simulink model "vector_vehicle_canoe"  (Simulink 7.7)
settings: Solver=ode3  StartTime=0.0  StopTime=10.0  FixedStep=T  RelTol=1e-3
libraries: canoelib x70, simulink x3
settings Model: Creator=vismso  LastModifiedBy=visjf
settings DataIOCC: SaveOutput=off  SignalLogging=off  SaveTime=off
settings OptimizationCC: InlineParams=on  UseIntDivNetSlope=on  SimCompilerOptimization=On
settings DebuggingCC: ArtificialAlgebraicLoopMsg=none  StrictBusMsg=Warning
settings RTWCC: SystemTargetFile=cn.tlc  TemplateMakefile=cn_msdll.tmf  Description=Vector CANoe Real-Time Target DLL (Visual C/C++ Project Makefile)  ProcessScript=cn_make_rtw_hook
settings CodeAppCC: MaxIdLength=128
settings STFCustomTargetCC: FunctionExecutionProfile=off  GeneratePreprocessorConditionals=Disable all  MatFileLogging=on  SystemTargetFile=cn.tlc
settings GRTTargetCC: ParMdlRefBuildCompliant=off  CompOptLevelCompliant=off  ExtModeMexFile=noextcomm  RTWCAPISignals=on  RTWCAPIParams=on
settings CustomProperty: DataType=string  Value=..\canoe

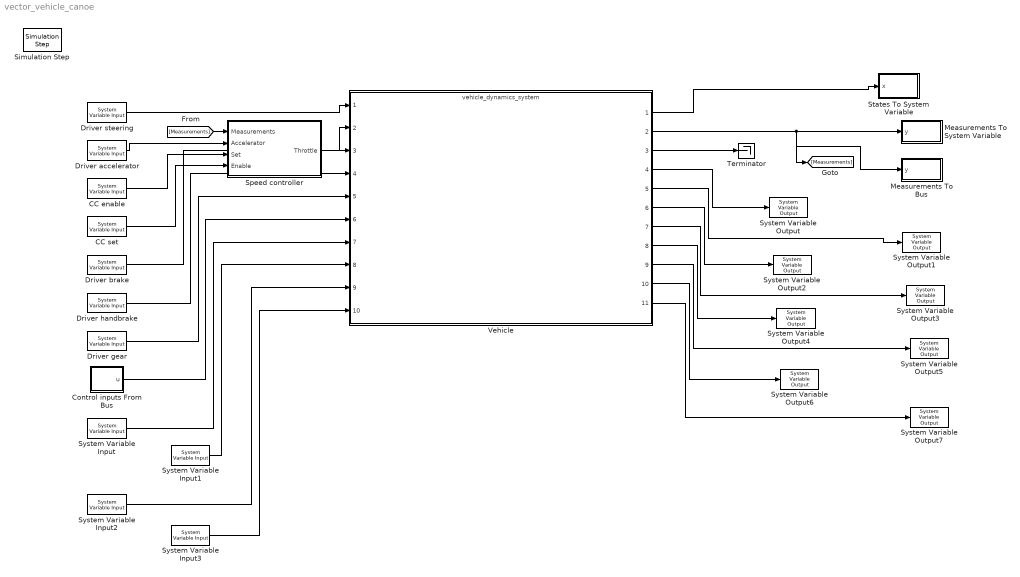
== system vector_vehicle_canoe ==
  CC enable : canoelib/CANoe I//O/System Variable Input  SystemSampleTime=-1  nsName=ModelStimuli  sysVarName=Crse_Ctrl_Set  arrayIndex=-1  editSampleTime=0
      settings: AttributesFormatString=%<nsName>::%<sysVarName>
  CC set : canoelib/CANoe I//O/System Variable Input  SystemSampleTime=-1  nsName=ModelStimuli  sysVarName=Crse_Ctrl_Enable  arrayIndex=-1  editSampleTime=0
      settings: AttributesFormatString=%<nsName>::%<sysVarName>
  Control inputs From Bus : Subsystem
  Driver accelerator : canoelib/CANoe I//O/System Variable Input  SystemSampleTime=-1  nsName=ModelStimuli  sysVarName=Driver_Accelerator  arrayIndex=-1  editSampleTime=0
      settings: AttributesFormatString=%<nsName>::%<sysVarName>
  Driver brake : canoelib/CANoe I//O/System Variable Input  SystemSampleTime=-1  nsName=ModelStimuli  sysVarName=Driver_Brake  arrayIndex=-1  editSampleTime=0
      settings: AttributesFormatString=%<nsName>::%<sysVarName>
  Driver gear : canoelib/CANoe I//O/System Variable Input  SystemSampleTime=-1  nsName=ModelStimuli  sysVarName=Driver_Gear  arrayIndex=-1  editSampleTime=0
      settings: AttributesFormatString=%<nsName>::%<sysVarName>
  Driver handbrake : canoelib/CANoe I//O/System Variable Input  SystemSampleTime=-1  nsName=ModelStimuli  sysVarName=Driver_Handbrake  arrayIndex=-1  editSampleTime=0
      settings: AttributesFormatString=%<nsName>::%<sysVarName>
  Driver steering : canoelib/CANoe I//O/System Variable Input  SystemSampleTime=-1  nsName=ModelStimuli  sysVarName=Driver_Steer  arrayIndex=-1  editSampleTime=0
      settings: AttributesFormatString=%<nsName>::%<sysVarName>
  Measurements To Bus : Subsystem
  Measurements To System Variable : Subsystem
  Simulation Step : canoelib/CANoe I//O/Simulation Step  SystemSampleTime=-1  mode=Synchronized
      settings: AttributesFormatString=%<mode>
  Speed controller : Subsystem  mask(Speed controller){vic=0/3.6}
      mask prompts: vic "Initial setpoint speed [m/s]"
      mask help:
      | This block forms a simple PI-controller for the vehicle forward speed.
      |
      | The "Enable" input enables the controller on any input greater than zero.
      | If disabled, the "Accelerator" signal is directly fed through towards the
      | vehicle's engine as "Throttle" signal.
      |
      | On a rising edge of "Set" the current forward velocity is taken as a
      | setpoint for the controller. Also, the current "Accelerator" value is taken
      | as initial value for the integral part of the PI-controller.
      mask Display: %image(imread('cruisecontrol.jpg'))
  States To System Variable : Subsystem
  System Variable Input : canoelib/CANoe I//O/System Variable Input  SystemSampleTime=-1  nsName=ModelDamperForces  sysVarName=DamperForceRR  arrayIndex=-1  editSampleTime=0
      settings: AttributesFormatString=%<nsName>::%<sysVarName>
  System Variable Input1 : canoelib/CANoe I//O/System Variable Input  SystemSampleTime=-1  nsName=ModelDamperForces  sysVarName=DamperForceRL  arrayIndex=-1  editSampleTime=0
      settings: AttributesFormatString=%<nsName>::%<sysVarName>
  System Variable Input2 : canoelib/CANoe I//O/System Variable Input  SystemSampleTime=-1  nsName=ModelDamperForces  sysVarName=DamperForceFR  arrayIndex=-1  editSampleTime=0
      settings: AttributesFormatString=%<nsName>::%<sysVarName>
  System Variable Input3 : canoelib/CANoe I//O/System Variable Input  SystemSampleTime=-1  nsName=ModelDamperForces  sysVarName=DamperForceFL  arrayIndex=-1  editSampleTime=0
      settings: AttributesFormatString=%<nsName>::%<sysVarName>
  System Variable Output : canoelib/CANoe I//O/System Variable Output  SystemSampleTime=-1  nsName=ModelDamper  sysVarName=Damper_RR_suspdeflection  arrayIndex=-1
      settings: AttributesFormatString=%<nsName>::%<sysVarName>
  System Variable Output1 : canoelib/CANoe I//O/System Variable Output  SystemSampleTime=-1  nsName=ModelDamper  sysVarName=Damper_RR1dot_suspvelocity  arrayIndex=-1
      settings: AttributesFormatString=%<nsName>::%<sysVarName>
  System Variable Output2 : canoelib/CANoe I//O/System Variable Output  SystemSampleTime=-1  nsName=ModelDamper  sysVarName=Damper_RL_suspdeflection  arrayIndex=-1
      settings: AttributesFormatString=%<nsName>::%<sysVarName>
  System Variable Output3 : canoelib/CANoe I//O/System Variable Output  SystemSampleTime=-1  nsName=ModelDamper  sysVarName=Damper_RL1dot_suspvelocity  arrayIndex=-1
      settings: AttributesFormatString=%<nsName>::%<sysVarName>
  System Variable Output4 : canoelib/CANoe I//O/System Variable Output  SystemSampleTime=-1  nsName=ModelDamper  sysVarName=Damper_FR_suspdeflection  arrayIndex=-1
      settings: AttributesFormatString=%<nsName>::%<sysVarName>
  System Variable Output5 : canoelib/CANoe I//O/System Variable Output  SystemSampleTime=-1  nsName=ModelDamper  sysVarName=Damper_FR1dot_suspvelocity  arrayIndex=-1
      settings: AttributesFormatString=%<nsName>::%<sysVarName>
  System Variable Output6 : canoelib/CANoe I//O/System Variable Output  SystemSampleTime=-1  nsName=ModelDamper  sysVarName=Damper_FL_suspdeflection  arrayIndex=-1
      settings: AttributesFormatString=%<nsName>::%<sysVarName>
  System Variable Output7 : canoelib/CANoe I//O/System Variable Output  SystemSampleTime=-1  nsName=ModelDamper  sysVarName=Damper_FL1dot_suspvelocity  arrayIndex=-1
      settings: AttributesFormatString=%<nsName>::%<sysVarName>
  Terminator : Terminator
  Vehicle : ModelReference  ModelNameDialog=vehicle_dynamics_system  SimulationMode=Normal  ModelReferenceVersion=1.93  CopyOfModelName=vehicle_dynamics_system  DefaultDataLogging=off
      mask init:
      | load_system(get(gcbh,'ModelName'));
      | 
      | inputs=find_system(get(gcbh,'ModelName'),'SearchDepth',1,'LookUnderMasks','on','BlockType','Inport');
      | outputs=find_system(get(gcbh,'ModelName'),'SearchDepth',1,'LookUnderMasks','on','BlockType','Outport');
      | 
      | for i = 1:length(inputs)
      |     s.(['inport' num2str(i)]) = str2num(get_param(inputs{i},'Port'));
      |     s.(['inname' num2str(i)]) = get_param(inputs{i},'Name');
      | end
      | 
      | for i = 1:length(outputs)
      |     s.(['outport' num2str(i)]) = str2num(get_param(outputs{i},'Port'));
      |     s.(['outname' num2str(i)]) = get_param(outputs{i},'Name');
      | end
      mask Display:
      | image(imread('vector_car.jpg'))
      | 
      | color('white')
      | 
      | port_label('input',s.inport1,s.inname1)
      | port_label('input',s.inport2,s.inname2)
      | port_label('input',s.inport3,s.inname3)
      | port_label('input',s.inport4,s.inname4)
      | port_label('input',s.inport5,s.inname5)
      | port_label('input',s.inport6,s.inname6)
      | 
      | port_label('output',s.outport1,s.outname1)
      | port_label('output',s.outport2,s.outname2)
      | port_label('output',s.outport3,s.outname3)
  wires:
  Driver gear/1 -> Vehicle/5
  Driver handbrake/1 -> Vehicle/4
  Driver brake/1 -> Vehicle/3
  Driver steering/1 -> Vehicle/1
  Control inputs From Bus/1(u) -> Vehicle/6
  Vehicle/2 -> Measurements To Bus/1(y), [Measurements], Measurements To System Variable/1(y)
  Vehicle/1 -> States To System Variable/1(x)
  Speed controller/1(Throttle) -> Vehicle/2
  [Measurements] -> Speed controller/1(Measurements)
  Driver accelerator/1 -> Speed controller/2(Accelerator)
  CC enable/1 -> Speed controller/3(Set)
  CC set/1 -> Speed controller/4(Enable)
  Vehicle/3 -> Terminator/1
  System Variable Input/1 -> Vehicle/7
  Vehicle/4 -> System Variable Output/1
  Vehicle/5 -> System Variable Output1/1
  Vehicle/6 -> System Variable Output2/1
  Vehicle/7 -> System Variable Output3/1
  Vehicle/8 -> System Variable Output4/1
  Vehicle/9 -> System Variable Output5/1
  Vehicle/10 -> System Variable Output6/1
  Vehicle/11 -> System Variable Output7/1
  System Variable Input1/1 -> Vehicle/8
  System Variable Input2/1 -> Vehicle/9
  System Variable Input3/1 -> Vehicle/10

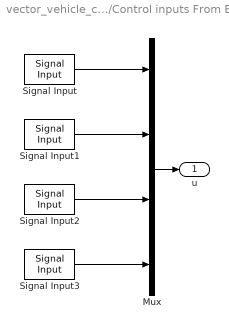
== system vector_vehicle_canoe/Control inputs From Bus ==
  Mux : Mux
  Signal Input : canoelib/CANoe I//O/Signal Input  SystemSampleTime=-1  dbName=""  nodeName=""  msgName=""  sigName=Susp_Ctrl_DesiredForce_FL  editSampleTime=0  rawValue=off
      settings: AttributesFormatString=%<sigName>
  Signal Input1 : canoelib/CANoe I//O/Signal Input  SystemSampleTime=-1  dbName=""  nodeName=""  msgName=""  sigName=Susp_Ctrl_DesiredForce_FR  editSampleTime=0  rawValue=off
      settings: AttributesFormatString=%<sigName>
  Signal Input2 : canoelib/CANoe I//O/Signal Input  SystemSampleTime=-1  dbName=""  nodeName=""  msgName=""  sigName=Susp_Ctrl_DesiredForce_RL  editSampleTime=0  rawValue=off
      settings: AttributesFormatString=%<sigName>
  Signal Input3 : canoelib/CANoe I//O/Signal Input  SystemSampleTime=-1  dbName=""  nodeName=""  msgName=""  sigName=Susp_Ctrl_DesiredForce_RR  editSampleTime=0  rawValue=off
      settings: AttributesFormatString=%<sigName>
  u : Outport
  wires:
  Signal Input/1 -> Mux/1
  Signal Input1/1 -> Mux/2
  Signal Input2/1 -> Mux/3
  Signal Input3/1 -> Mux/4
  Mux/1 -> u/1

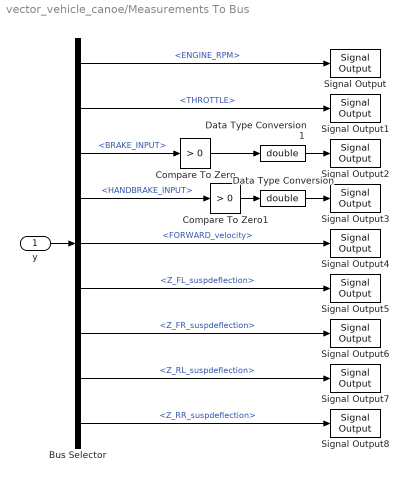
== system vector_vehicle_canoe/Measurements To Bus ==
  y : Inport
  Bus Selector : BusSelector  OutputSignals=ENGINE_RPM,THROTTLE,BRAKE_INPUT,HANDBRAKE_INPUT,FORWARD_velocity,Z_FL_suspdeflection,Z_FR_suspdeflection,Z_RL_suspdeflection,Z_RR_suspdeflection
  Compare To Zero : simulink/Logic and Bit Operations/Compare To Zero  SystemSampleTime=-1  relop=>  LogicOutDataTypeMode=uint8
  Compare To Zero1 : simulink/Logic and Bit Operations/Compare To Zero  SystemSampleTime=-1  relop=>  LogicOutDataTypeMode=uint8
  Data Type Conversion : DataTypeConversion  OutDataTypeStr=double
  Data Type Conversion1 : DataTypeConversion  OutDataTypeStr=double
  Signal Output : canoelib/CANoe I//O/Signal Output  SystemSampleTime=-1  dbName=""  nodeName=""  msgName=""  sigName=Eng_RPM  rawValue=off
      settings: AttributesFormatString=%<sigName>
  Signal Output1 : canoelib/CANoe I//O/Signal Output  SystemSampleTime=-1  dbName=""  nodeName=""  msgName=""  sigName=Eng_Throttle  rawValue=off
      settings: AttributesFormatString=%<sigName>
  Signal Output2 : canoelib/CANoe I//O/Signal Output  SystemSampleTime=-1  dbName=""  nodeName=""  msgName=""  sigName=Vehicle_BrakePedal  rawValue=off
      settings: AttributesFormatString=%<sigName>
  Signal Output3 : canoelib/CANoe I//O/Signal Output  SystemSampleTime=-1  dbName=""  nodeName=""  msgName=""  sigName=Vehicle_Handbrake  rawValue=off
      settings: AttributesFormatString=%<sigName>
  Signal Output4 : canoelib/CANoe I//O/Signal Output  SystemSampleTime=-1  dbName=""  nodeName=""  msgName=""  sigName=Vehicle_ForwardSpeed  rawValue=off
      settings: AttributesFormatString=%<sigName>
  Signal Output5 : canoelib/CANoe I//O/Signal Output  SystemSampleTime=-1  dbName=""  nodeName=""  msgName=""  sigName=Susp_Ctrl_SuspDefl_FL  rawValue=off
      settings: AttributesFormatString=%<sigName>
  Signal Output6 : canoelib/CANoe I//O/Signal Output  SystemSampleTime=-1  dbName=""  nodeName=""  msgName=""  sigName=Susp_Ctrl_SuspDefl_FR  rawValue=off
      settings: AttributesFormatString=%<sigName>
  Signal Output7 : canoelib/CANoe I//O/Signal Output  SystemSampleTime=-1  dbName=""  nodeName=""  msgName=""  sigName=Susp_Ctrl_SuspDefl_RL  rawValue=off
      settings: AttributesFormatString=%<sigName>
  Signal Output8 : canoelib/CANoe I//O/Signal Output  SystemSampleTime=-1  dbName=""  nodeName=""  msgName=""  sigName=Susp_Ctrl_SuspDefl_RR  rawValue=off
      settings: AttributesFormatString=%<sigName>
  wires:
  y/1 -> Bus Selector/1
  Bus Selector/1 -> Signal Output/1  "<ENGINE_RPM>"
  Bus Selector/2 -> Signal Output1/1  "<THROTTLE>"
  Bus Selector/3 -> Compare To Zero/1  "<BRAKE_INPUT>"
  Bus Selector/4 -> Compare To Zero1/1  "<HANDBRAKE_INPUT>"
  Bus Selector/5 -> Signal Output4/1  "<FORWARD_velocity>"
  Compare To Zero/1 -> Data Type Conversion1/1
  Compare To Zero1/1 -> Data Type Conversion/1
  Data Type Conversion/1 -> Signal Output3/1
  Data Type Conversion1/1 -> Signal Output2/1
  Bus Selector/6 -> Signal Output5/1  "<Z_FL_suspdeflection>"
  Bus Selector/7 -> Signal Output6/1  "<Z_FR_suspdeflection>"
  Bus Selector/8 -> Signal Output7/1  "<Z_RL_suspdeflection>"
  Bus Selector/9 -> Signal Output8/1  "<Z_RR_suspdeflection>"

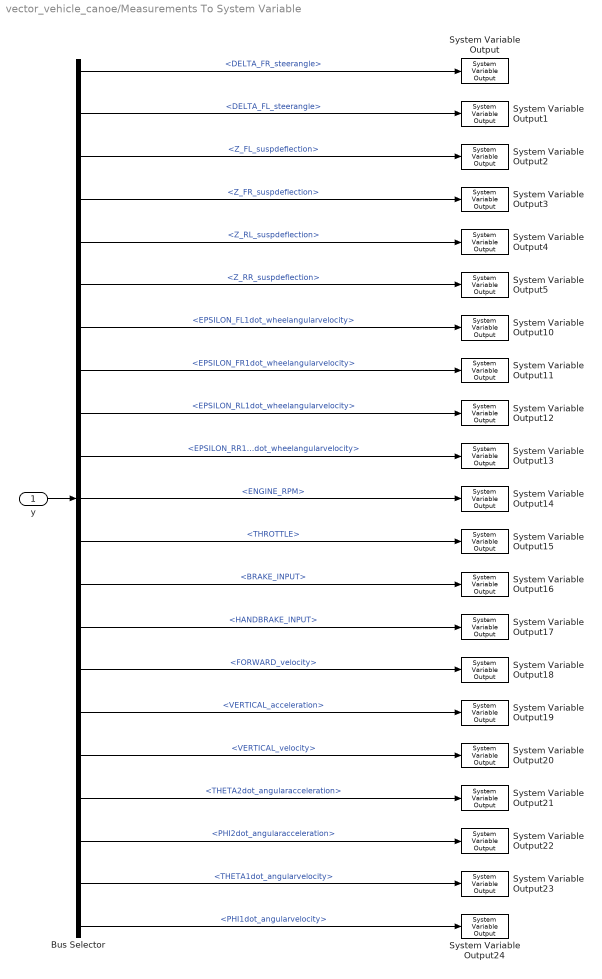
== system vector_vehicle_canoe/Measurements To System Variable ==
  y : Inport
  Bus Selector : BusSelector  OutputSignals=DELTA_FR_steerangle,DELTA_FL_steerangle,Z_FL_suspdeflection,Z_FR_suspdeflection,Z_RL_suspdeflection,Z_RR_suspdeflection,EPSILON_FL1dot_wheelangularvelocity,EPSILON_FR1dot_wheelangularvelocity,EPSILON_RL1dot_wheelangularvelocity,EPSILON_RR1dot_wheelangularvelocity,ENGINE_RPM,THROTTLE,BRAKE_INPUT,HANDBRAKE_INPUT,FORWARD_velocity,VERTICAL_acceleration,VERTICAL_velocity,THETA2dot_angularacceleration,PHI2dot_angularacceleration,THETA1dot_angularvelocity,PHI1dot_angularvelocity
  System Variable Output : canoelib/CANoe I//O/System Variable Output  SystemSampleTime=-1  nsName=ModelLocalMeasurements  sysVarName=SteerAngleFL  arrayIndex=-1
      settings: AttributesFormatString=%<nsName>::%<sysVarName>
  System Variable Output1 : canoelib/CANoe I//O/System Variable Output  SystemSampleTime=-1  nsName=ModelLocalMeasurements  sysVarName=SteerAngleFR  arrayIndex=-1
      settings: AttributesFormatString=%<nsName>::%<sysVarName>
  System Variable Output10 : canoelib/CANoe I//O/System Variable Output  SystemSampleTime=-1  nsName=ModelLocalMeasurements  sysVarName=WheelSpeedFL  arrayIndex=-1
      settings: AttributesFormatString=%<nsName>::%<sysVarName>
  System Variable Output11 : canoelib/CANoe I//O/System Variable Output  SystemSampleTime=-1  nsName=ModelLocalMeasurements  sysVarName=WheelSpeedFR  arrayIndex=-1
      settings: AttributesFormatString=%<nsName>::%<sysVarName>
  System Variable Output12 : canoelib/CANoe I//O/System Variable Output  SystemSampleTime=-1  nsName=ModelLocalMeasurements  sysVarName=WheelSpeedRL  arrayIndex=-1
      settings: AttributesFormatString=%<nsName>::%<sysVarName>
  System Variable Output13 : canoelib/CANoe I//O/System Variable Output  SystemSampleTime=-1  nsName=ModelLocalMeasurements  sysVarName=WheelSpeedRR  arrayIndex=-1
      settings: AttributesFormatString=%<nsName>::%<sysVarName>
  System Variable Output14 : canoelib/CANoe I//O/System Variable Output  SystemSampleTime=-1  nsName=ModelLocalMeasurements  sysVarName=EngineRPM  arrayIndex=-1
      settings: AttributesFormatString=%<nsName>::%<sysVarName>
  System Variable Output15 : canoelib/CANoe I//O/System Variable Output  SystemSampleTime=-1  nsName=ModelLocalMeasurements  sysVarName=Throttle  arrayIndex=-1
      settings: AttributesFormatString=%<nsName>::%<sysVarName>
  System Variable Output16 : canoelib/CANoe I//O/System Variable Output  SystemSampleTime=-1  nsName=ModelLocalMeasurements  sysVarName=Brake  arrayIndex=-1
      settings: AttributesFormatString=%<nsName>::%<sysVarName>
  System Variable Output17 : canoelib/CANoe I//O/System Variable Output  SystemSampleTime=-1  nsName=ModelLocalMeasurements  sysVarName=Handbrake  arrayIndex=-1
      settings: AttributesFormatString=%<nsName>::%<sysVarName>
  System Variable Output18 : canoelib/CANoe I//O/System Variable Output  SystemSampleTime=-1  nsName=ModelLocalMeasurements  sysVarName=ForwardVelocity  arrayIndex=-1
      settings: AttributesFormatString=%<nsName>::%<sysVarName>
  System Variable Output19 : canoelib/CANoe I//O/System Variable Output  SystemSampleTime=-1  nsName=ModelLocalMeasurements  sysVarName=BodyVerticalAcc  arrayIndex=-1
      settings: AttributesFormatString=%<nsName>::%<sysVarName>
  System Variable Output2 : canoelib/CANoe I//O/System Variable Output  SystemSampleTime=-1  nsName=ModelLocalMeasurements  sysVarName=SuspDeflectionFL  arrayIndex=-1
      settings: AttributesFormatString=%<nsName>::%<sysVarName>
  System Variable Output20 : canoelib/CANoe I//O/System Variable Output  SystemSampleTime=-1  nsName=ModelLocalMeasurements  sysVarName=BodyVerticalVel  arrayIndex=-1
      settings: AttributesFormatString=%<nsName>::%<sysVarName>
  System Variable Output21 : canoelib/CANoe I//O/System Variable Output  SystemSampleTime=-1  nsName=ModelLocalMeasurements  sysVarName=BodyPitchAcc  arrayIndex=-1
      settings: AttributesFormatString=%<nsName>::%<sysVarName>
  System Variable Output22 : canoelib/CANoe I//O/System Variable Output  SystemSampleTime=-1  nsName=ModelLocalMeasurements  sysVarName=BodyRollAcc  arrayIndex=-1
      settings: AttributesFormatString=%<nsName>::%<sysVarName>
  System Variable Output23 : canoelib/CANoe I//O/System Variable Output  SystemSampleTime=-1  nsName=ModelLocalMeasurements  sysVarName=BodyPitchVel  arrayIndex=-1
      settings: AttributesFormatString=%<nsName>::%<sysVarName>
  System Variable Output24 : canoelib/CANoe I//O/System Variable Output  SystemSampleTime=-1  nsName=ModelLocalMeasurements  sysVarName=BodyRollVel  arrayIndex=-1
      settings: AttributesFormatString=%<nsName>::%<sysVarName>
  System Variable Output3 : canoelib/CANoe I//O/System Variable Output  SystemSampleTime=-1  nsName=ModelLocalMeasurements  sysVarName=SuspDeflectionFR  arrayIndex=-1
      settings: AttributesFormatString=%<nsName>::%<sysVarName>
  System Variable Output4 : canoelib/CANoe I//O/System Variable Output  SystemSampleTime=-1  nsName=ModelLocalMeasurements  sysVarName=SuspDeflectionRL  arrayIndex=-1
      settings: AttributesFormatString=%<nsName>::%<sysVarName>
  System Variable Output5 : canoelib/CANoe I//O/System Variable Output  SystemSampleTime=-1  nsName=ModelLocalMeasurements  sysVarName=SuspDeflectionRR  arrayIndex=-1
      settings: AttributesFormatString=%<nsName>::%<sysVarName>
  wires:
  y/1 -> Bus Selector/1
  Bus Selector/1 -> System Variable Output/1  "<DELTA_FR_steerangle>"
  Bus Selector/2 -> System Variable Output1/1  "<DELTA_FL_steerangle>"
  Bus Selector/3 -> System Variable Output2/1  "<Z_FL_suspdeflection>"
  Bus Selector/4 -> System Variable Output3/1  "<Z_FR_suspdeflection>"
  Bus Selector/5 -> System Variable Output4/1  "<Z_RL_suspdeflection>"
  Bus Selector/6 -> System Variable Output5/1  "<Z_RR_suspdeflection>"
  Bus Selector/7 -> System Variable Output10/1  "<EPSILON_FL1dot_wheelangularvelocity>"
  Bus Selector/8 -> System Variable Output11/1  "<EPSILON_FR1dot_wheelangularvelocity>"
  Bus Selector/9 -> System Variable Output12/1  "<EPSILON_RL1dot_wheelangularvelocity>"
  Bus Selector/10 -> System Variable Output13/1  "<EPSILON_RR1dot_wheelangularvelocity>"
  Bus Selector/11 -> System Variable Output14/1  "<ENGINE_RPM>"
  Bus Selector/12 -> System Variable Output15/1  "<THROTTLE>"
  Bus Selector/13 -> System Variable Output16/1  "<BRAKE_INPUT>"
  Bus Selector/14 -> System Variable Output17/1  "<HANDBRAKE_INPUT>"
  Bus Selector/15 -> System Variable Output18/1  "<FORWARD_velocity>"
  Bus Selector/16 -> System Variable Output19/1  "<VERTICAL_acceleration>"
  Bus Selector/17 -> System Variable Output20/1  "<VERTICAL_velocity>"
  Bus Selector/18 -> System Variable Output21/1  "<THETA2dot_angularacceleration>"
  Bus Selector/19 -> System Variable Output22/1  "<PHI2dot_angularacceleration>"
  Bus Selector/20 -> System Variable Output23/1  "<THETA1dot_angularvelocity>"
  Bus Selector/21 -> System Variable Output24/1  "<PHI1dot_angularvelocity>"

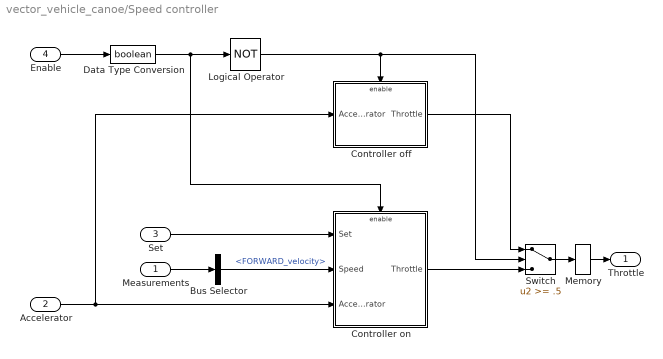
== system vector_vehicle_canoe/Speed controller ==
  Measurements : Inport
  Accelerator : Inport  Port=2
  Set : Inport  Port=3
  Enable : Inport  Port=4
  Bus Selector : BusSelector  OutputSignals=FORWARD_velocity
  Controller off : Subsystem
  Controller on : Subsystem
  Data Type Conversion : DataTypeConversion  OutDataTypeStr=boolean
  Logical Operator : Logic  Operator=NOT  AllPortsSameDT=off  OutDataTypeStr=boolean
  Memory : Memory
  Switch : Switch  Threshold=.5
  Throttle : Outport
  wires:
  Measurements/1 -> Bus Selector/1
  Accelerator/1 -> Controller on/3(Accelerator), Controller off/1(Accelerator)
  Set/1 -> Controller on/1(Set)
  Bus Selector/1 -> Controller on/2(Speed)  "<FORWARD_velocity>"
  Switch/1 -> Memory/1
  Enable/1 -> Data Type Conversion/1
  Logical Operator/1 -> Controller off/Enable, Switch/2
  Controller off/1(Throttle) -> Switch/1
  Controller on/1(Throttle) -> Switch/3
  Data Type Conversion/1 -> Logical Operator/1, Controller on/Enable
  Memory/1 -> Throttle/1

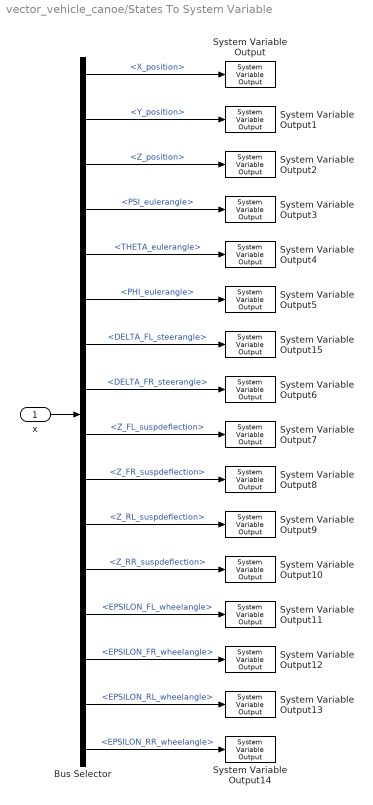
== system vector_vehicle_canoe/States To System Variable ==
  x : Inport
  Bus Selector : BusSelector  OutputSignals=X_position,Y_position,Z_position,PSI_eulerangle,THETA_eulerangle,PHI_eulerangle,DELTA_FL_steerangle,DELTA_FR_steerangle,Z_FL_suspdeflection,Z_FR_suspdeflection,Z_RL_suspdeflection,Z_RR_suspdeflection,EPSILON_FL_wheelangle,EPSILON_FR_wheelangle,EPSILON_RL_wheelangle,EPSILON_RR_wheelangle
  System Variable Output : canoelib/CANoe I//O/System Variable Output  SystemSampleTime=-1  nsName=ModelStates  sysVarName=VehicleStates  arrayIndex=0
      settings: AttributesFormatString=%<nsName>::%<sysVarName>[%<arrayIndex>]
  System Variable Output1 : canoelib/CANoe I//O/System Variable Output  SystemSampleTime=-1  nsName=ModelStates  sysVarName=VehicleStates  arrayIndex=1
      settings: AttributesFormatString=%<nsName>::%<sysVarName>[%<arrayIndex>]
  System Variable Output10 : canoelib/CANoe I//O/System Variable Output  SystemSampleTime=-1  nsName=ModelStates  sysVarName=VehicleStates  arrayIndex=11
      settings: AttributesFormatString=%<nsName>::%<sysVarName>[%<arrayIndex>]
  System Variable Output11 : canoelib/CANoe I//O/System Variable Output  SystemSampleTime=-1  nsName=ModelStates  sysVarName=VehicleStates  arrayIndex=12
      settings: AttributesFormatString=%<nsName>::%<sysVarName>[%<arrayIndex>]
  System Variable Output12 : canoelib/CANoe I//O/System Variable Output  SystemSampleTime=-1  nsName=ModelStates  sysVarName=VehicleStates  arrayIndex=13
      settings: AttributesFormatString=%<nsName>::%<sysVarName>[%<arrayIndex>]
  System Variable Output13 : canoelib/CANoe I//O/System Variable Output  SystemSampleTime=-1  nsName=ModelStates  sysVarName=VehicleStates  arrayIndex=14
      settings: AttributesFormatString=%<nsName>::%<sysVarName>[%<arrayIndex>]
  System Variable Output14 : canoelib/CANoe I//O/System Variable Output  SystemSampleTime=-1  nsName=ModelStates  sysVarName=VehicleStates  arrayIndex=15
      settings: AttributesFormatString=%<nsName>::%<sysVarName>[%<arrayIndex>]
  System Variable Output15 : canoelib/CANoe I//O/System Variable Output  SystemSampleTime=-1  nsName=ModelStates  sysVarName=VehicleStates  arrayIndex=6
      settings: AttributesFormatString=%<nsName>::%<sysVarName>[%<arrayIndex>]
  System Variable Output2 : canoelib/CANoe I//O/System Variable Output  SystemSampleTime=-1  nsName=ModelStates  sysVarName=VehicleStates  arrayIndex=2
      settings: AttributesFormatString=%<nsName>::%<sysVarName>[%<arrayIndex>]
  System Variable Output3 : canoelib/CANoe I//O/System Variable Output  SystemSampleTime=-1  nsName=ModelStates  sysVarName=VehicleStates  arrayIndex=3
      settings: AttributesFormatString=%<nsName>::%<sysVarName>[%<arrayIndex>]
  System Variable Output4 : canoelib/CANoe I//O/System Variable Output  SystemSampleTime=-1  nsName=ModelStates  sysVarName=VehicleStates  arrayIndex=4
      settings: AttributesFormatString=%<nsName>::%<sysVarName>[%<arrayIndex>]
  System Variable Output5 : canoelib/CANoe I//O/System Variable Output  SystemSampleTime=-1  nsName=ModelStates  sysVarName=VehicleStates  arrayIndex=5
      settings: AttributesFormatString=%<nsName>::%<sysVarName>[%<arrayIndex>]
  System Variable Output6 : canoelib/CANoe I//O/System Variable Output  SystemSampleTime=-1  nsName=ModelStates  sysVarName=VehicleStates  arrayIndex=7
      settings: AttributesFormatString=%<nsName>::%<sysVarName>[%<arrayIndex>]
  System Variable Output7 : canoelib/CANoe I//O/System Variable Output  SystemSampleTime=-1  nsName=ModelStates  sysVarName=VehicleStates  arrayIndex=8
      settings: AttributesFormatString=%<nsName>::%<sysVarName>[%<arrayIndex>]
  System Variable Output8 : canoelib/CANoe I//O/System Variable Output  SystemSampleTime=-1  nsName=ModelStates  sysVarName=VehicleStates  arrayIndex=9
      settings: AttributesFormatString=%<nsName>::%<sysVarName>[%<arrayIndex>]
  System Variable Output9 : canoelib/CANoe I//O/System Variable Output  SystemSampleTime=-1  nsName=ModelStates  sysVarName=VehicleStates  arrayIndex=10
      settings: AttributesFormatString=%<nsName>::%<sysVarName>[%<arrayIndex>]
  wires:
  x/1 -> Bus Selector/1
  Bus Selector/1 -> System Variable Output/1  "<X_position>"
  Bus Selector/2 -> System Variable Output1/1  "<Y_position>"
  Bus Selector/3 -> System Variable Output2/1  "<Z_position>"
  Bus Selector/4 -> System Variable Output3/1  "<PSI_eulerangle>"
  Bus Selector/5 -> System Variable Output4/1  "<THETA_eulerangle>"
  Bus Selector/6 -> System Variable Output5/1  "<PHI_eulerangle>"
  Bus Selector/7 -> System Variable Output15/1  "<DELTA_FL_steerangle>"
  Bus Selector/8 -> System Variable Output6/1  "<DELTA_FR_steerangle>"
  Bus Selector/9 -> System Variable Output7/1  "<Z_FL_suspdeflection>"
  Bus Selector/10 -> System Variable Output8/1  "<Z_FR_suspdeflection>"
  Bus Selector/11 -> System Variable Output9/1  "<Z_RL_suspdeflection>"
  Bus Selector/12 -> System Variable Output10/1  "<Z_RR_suspdeflection>"
  Bus Selector/13 -> System Variable Output11/1  "<EPSILON_FL_wheelangle>"
  Bus Selector/14 -> System Variable Output12/1  "<EPSILON_FR_wheelangle>"
  Bus Selector/15 -> System Variable Output13/1  "<EPSILON_RL_wheelangle>"
  Bus Selector/16 -> System Variable Output14/1  "<EPSILON_RR_wheelangle>"

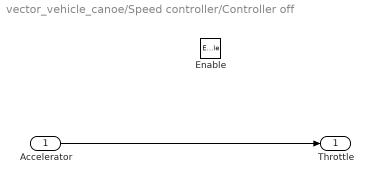
== system vector_vehicle_canoe/Speed controller/Controller off ==
  Accelerator : Inport
  Enable : EnablePort
  Throttle : Outport
  wires:
  Accelerator/1 -> Throttle/1

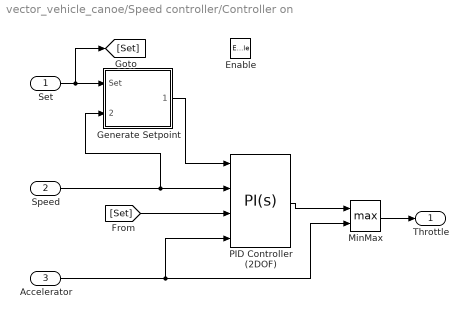
== system vector_vehicle_canoe/Speed controller/Controller on ==
  Set : Inport
  Speed : Inport  Port=2
  Accelerator : Inport  Port=3
  Enable : EnablePort
  Generate Setpoint : Subsystem
  MinMax : MinMax  Function=max  Inputs=2
  PID Controller (2DOF) : simulink/Continuous/PID Controller (2DOF)  SystemSampleTime=-1  Controller=PI  TimeDomain=Continuous-time  SampleTime=1  IntegratorMethod=Forward Euler  FilterMethod=Forward Euler  Form=Parallel  P=1  I=1  D=0  N=100  b=1  c=1  InitialConditionSource=external  InitialConditionForIntegrator=0  InitialConditionForFilter=0  ExternalReset=rising  LimitOutput=on  UpperSaturationLimit=1  LowerSaturationLimit=0  LinearizeAsGain=off  AntiWindupMode=clamping  Kb=1  TrackingMode=off  Kt=1  PParamMin=[]  PParamMax=[]  IParamMin=[]  IParamMax=[]  DParamMin=[]  DParamMax=[]  NParamMin=[]  NParamMax=[]  bParamMin=[]  bParamMax=[]  cParamMin=[]  cParamMax=[]  KbParamMin=[]  KbParamMax=[]  KtParamMin=[]  KtParamMax=[]  POutMin=[]  POutMax=[]  IOutMin=[]  IOutMax=[]  DOutMin=[]  DOutMax=[]  NOutMin=[]  NOutMax=[]  bOutMin=[]  bOutMax=[]  cOutMin=[]  cOutMax=[]  KbOutMin=[]  KbOutMax=[]  KtOutMin=[]  KtOutMax=[]  IntegratorOutMin=[]  IntegratorOutMax=[]  FilterOutMin=[]  FilterOutMax=[]  SumOutMin=[]  SumOutMax=[]  Sum1OutMin=[]  Sum1OutMax=[]  Sum2OutMin=[]  Sum2OutMax=[]  Sum3OutMin=[]  Sum3OutMax=[]  SumI1OutMin=[]  SumI1OutMax=[]  SumI2OutMin=[]  SumI2OutMax=[]  SumI3OutMin=[]  SumI3OutMax=[]  SumDOutMin=[]  SumDOutMax=[]  SaturationOutMin=[]  SaturationOutMax=[]  IntegratorContinuousStateAttributes=''  IntegratorStateMustResolveToSignalObject=off  IntegratorRTWStateStorageClass=Auto  FilterContinuousStateAttributes=''  FilterStateMustResolveToSignalObject=off  FilterRTWStateStorageClass=Auto
  Throttle : Outport
  wires:
  PID Controller (2DOF)/1 -> MinMax/1
  Generate Setpoint/1(Setpoint) -> PID Controller (2DOF)/1
  Set/1 -> Generate Setpoint/1(Set), [Set]
  Speed/1 -> Generate Setpoint/2(Speed), PID Controller (2DOF)/2
  MinMax/1 -> Throttle/1
  Accelerator/1 -> MinMax/2, PID Controller (2DOF)/4
  [Set] -> PID Controller (2DOF)/3

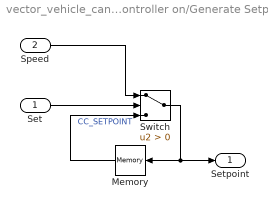
== system vector_vehicle_canoe/Speed controller/Controller on/Generate Setpoint ==
  Set : Inport
  Speed : Inport  Port=2
  Memory : Memory  X0=vic
  Switch : Switch  Criteria=u2 > Threshold
  Setpoint : Outport
  wires:
  Memory/1 -> Switch/3  "CC_SETPOINT"
  Switch/1 -> Memory/1, Setpoint/1
  Speed/1 -> Switch/1
  Set/1 -> Switch/2
